simulink model "rtwdemo_logicalORsf"  (Simulink 7.1)
settings: Solver=FixedStepDiscrete  StartTime=0.0  StopTime=10.0  RelTol=1e-3
PostLoadFcn:
  | load logicalOR.mat;
settings Model: Creator=ajayaram  LastModifiedBy=ajayaram
settings OptimizationCC: OptimizeModelRefInitCode=on  LifeSpan=1
settings RTWCC: SystemTargetFile=ert.tlc  GenCodeOnly=on  GenerateMakefile=off  TemplateMakefile=ert_default_tmf  Description=Real-Time Workshop Embedded Coder (no auto configuration)  GenerateReport=on  ProcessScript=ert_make_rtw_hook  IncludeHyperlinkInReport=on  LaunchReport=on
settings CodeAppCC: IgnoreCustomStorageClasses=off
settings ERTTargetCC: GenerateSampleERTMain=on  InlinedParameterPlacement=NonHierarchical  ERTCustomFileTemplate=example_file_process.tlc

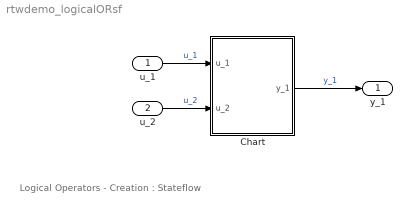
== system rtwdemo_logicalORsf ==
  note: Logical Operators - Creation : Stateflow
  u_1 : Inport  DataType=boolean  OutDataType=sfix(16)  OutScaling=2^0  OutDataTypeStr=boolean
  u_2 : Inport  Port=2  DataType=boolean  OutDataType=sfix(16)  OutScaling=2^0  OutDataTypeStr=boolean
  Chart : Stateflow chart
  y_1 : Outport  OutDataType=sfix(16)  OutScaling=2^0
  wires:
  u_1/1 -> Chart/1(u_1)  "u_1"
  u_2/1 -> Chart/2(u_2)  "u_2"
  Chart/1(y_1) -> y_1/1  "y_1"

== stateflow chart Chart ==
  (default) -> (junction 3)
  (junction 3) -> (junction 4) : {
      |  y_1 = u_1 || u_2 ;
      | }
  data: u_1 input boolean; u_2 input boolean; y_1 output boolean
